simulink model "HA2_Active_Body_Control_stud"  (R2016a)
settings: Solver=VariableStepAuto  StartTime=0.0  StopTime=10  FixedStep=0.01  RelTol=1e-3
values from neighbouring files (symbols this model uses):
  A_cyl = pi*(D_kolben^2)/4    (= 0.000314159265359)    [Active_Body_Control_param_stud.m]
  alpha_K_va = 0.6    [Active_Body_Control_param_stud.m]
  bore_max = 20e-6    (= 2e-05)    [Active_Body_Control_param_stud.m]
  c_A = 19000    [Active_Body_Control_param_stud.m]
  c_R = 190500    [Active_Body_Control_param_stud.m]
  d = 59    [Active_Body_Control_param_stud.m]
  d_A = 1100    [Active_Body_Control_param_stud.m]
  delta_y_s = 0.005    [Active_Body_Control_param_stud.m]
  g = 9.81    [Active_Body_Control_param_stud.m]
  Km = 1    [Active_Body_Control_param_stud.m]
  L = 1e-5    (= 1e-05)    [Active_Body_Control_param_stud.m]
  m_A = 200    [Active_Body_Control_param_stud.m]
  m_R = 40    [Active_Body_Control_param_stud.m]
  m_va = 0.1    [Active_Body_Control_param_stud.m]
  P_pump = 150e5    (= 15000000)    [Active_Body_Control_param_stud.m]
  R = 1.2    [Active_Body_Control_param_stud.m]
  rho = 880    [Active_Body_Control_param_stud.m]
  s_max_va = 0.020    (= 0.02)    [Active_Body_Control_param_stud.m]
settings Model: Creator=da.klinder  LastModifiedBy=Jason
settings DataIOCC: LimitDataPoints=on  SaveFormat=Array  SignalLoggingSaveFormat=ModelDataLogs
settings OptimizationCC: ExpressionDepthLimit=2147483647
settings DebuggingCC: UnderspecifiedInitializationDetection=Classic  MergeDetectMultiDrivingBlocksExec=none  SolverPrmCheckMsg=warning  FcnCallInpInsideContextMsg=EnableAllAsWarning  StateNameClashWarn=warning
settings HardwareCC: ProdBitPerPointer=32  ProdLargestAtomicFloat=None  ProdIntDivRoundTo=Undefined  ProdEndianess=Unspecified  ProdWordSize=32  ProdHWDeviceType=32-bit Generic
settings ModelReferenceCC: PropagateSignalLabelsOutOfModel=off
settings GRTTargetCC: CombineOutputUpdateFcns=off  GRTInterface=on

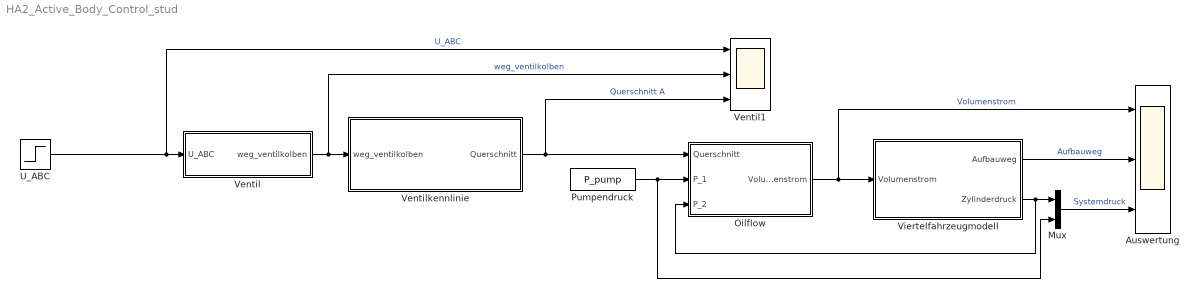
== system HA2_Active_Body_Control_stud ==
  Auswertung : Scope  NumInputPorts=3
  Mux : Mux  Inputs=2
  Oilflow : Subsystem
  Pumpendruck : Constant  Value=P_pump
  U_ABC : Step  Before=1  After=-1  SampleTime=0
  Ventil : Subsystem
  Ventil1 : Scope  NumInputPorts=3
  Ventilkennlinie : Subsystem
  Viertelfahrzeugmodell : Subsystem
  wires:
  Ventil/1(weg_ventilkolben) -> Ventilkennlinie/1(weg_ventilkolben), Ventil1/2  "weg_ventilkolben"
  Pumpendruck/1 -> Mux/2, Oilflow/2(P_1)
  Ventilkennlinie/1(Querschnitt) -> Ventil1/3, Oilflow/1(Querschnitt)  "Querschnitt A"
  Oilflow/1(Volumenstrom) -> Auswertung/1, Viertelfahrzeugmodell/1(Volumenstrom)  "Volumenstrom"
  Viertelfahrzeugmodell/2(Zylinderdruck) -> Mux/1, Oilflow/3(P_2)
  Mux/1 -> Auswertung/3  "Systemdruck"
  U_ABC/1 -> Ventil1/1, Ventil/1(U_ABC)  "U_ABC"
  Viertelfahrzeugmodell/1(Aufbauweg) -> Auswertung/2  "Aufbauweg"

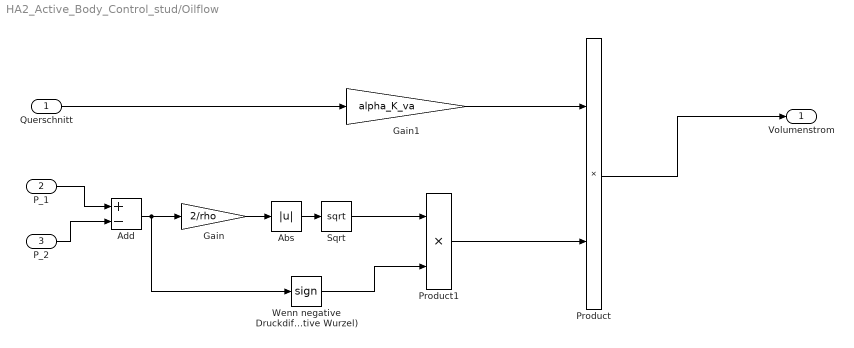
== system HA2_Active_Body_Control_stud/Oilflow ==
  Querschnitt : Inport
  P_1 : Inport  Port=2
  P_2 : Inport  Port=3
  Abs : Abs
  Add : Sum  Inputs=+-
  Gain : Gain  Gain=2/rho
  Gain1 : Gain  Gain=alpha_K_va
  Product : Product
  Product1 : Product
  Sqrt : Sqrt  SaturateOnIntegerOverflow=on
  "Wenn negative Druckdifferenz, dann auch negativer Volumenstrom (verhindert negative Wurzel)" : Signum
  Volumenstrom : Outport
  wires:
  P_1/1 -> Add/1
  P_2/1 -> Add/2
  Add/1 -> "Wenn negative Druckdifferenz, dann auch negativer Volumenstrom (verhindert negative Wurzel)"/1, Gain/1
  Gain/1 -> Abs/1
  Querschnitt/1 -> Gain1/1
  Product/1 -> Volumenstrom/1
  Abs/1 -> Sqrt/1
  Gain1/1 -> Product/1
  Sqrt/1 -> Product1/1
  "Wenn negative Druckdifferenz, dann auch negativer Volumenstrom (verhindert negative Wurzel)"/1 -> Product1/2
  Product1/1 -> Product/2

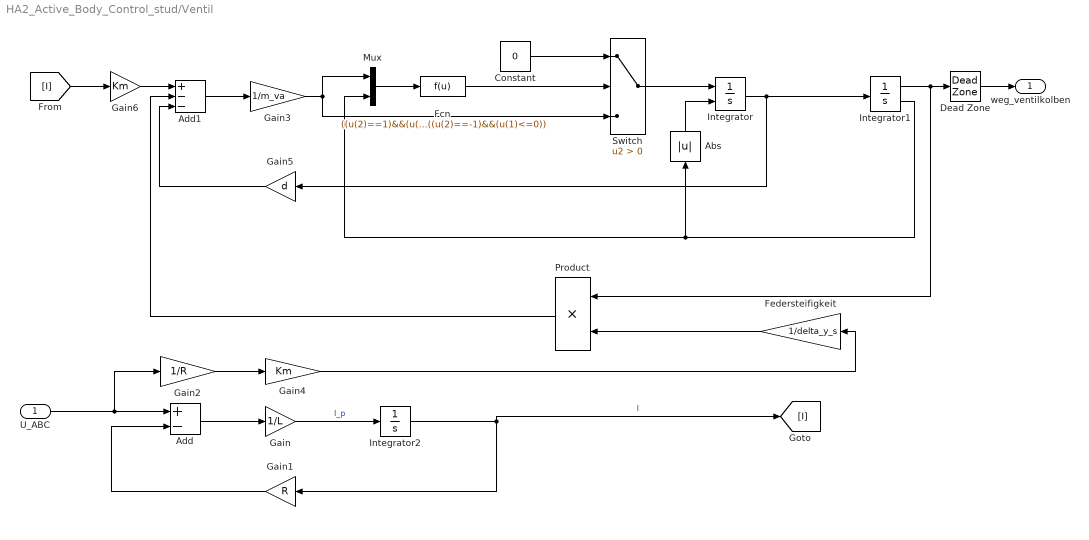
== system HA2_Active_Body_Control_stud/Ventil ==
  U_ABC : Inport
  Abs : Abs
  Add : Sum  Inputs=+-
  Add1 : Sum  Inputs=+--
  Constant : Constant  Value=0
  Dead Zone : DeadZone  SaturateOnIntegerOverflow=on
  Fcn : Fcn  Expr=((u(2)==1)&&(u(1)>=0))||((u(2)==-1)&&(u(1)<=0))
  Federsteifigkeit : Gain  Gain=1/delta_y_s
  Gain : Gain  Gain=1/L
  Gain1 : Gain  Gain=R
  Gain2 : Gain  Gain=1/R
  Gain3 : Gain  Gain=1/m_va
  Gain4 : Gain  Gain=Km
  Gain5 : Gain  Gain=d
  Gain6 : Gain  Gain=Km
  Integrator : Integrator  ExternalReset=rising
  Integrator1 : Integrator  LimitOutput=on  UpperSaturationLimit=s_max_va  LowerSaturationLimit=-s_max_va  ShowSaturationPort=on
  Integrator2 : Integrator
  Mux : Mux  Inputs=2
  Product : Product
  Switch : Switch  Criteria=u2 > Threshold
  weg_ventilkolben : Outport
  wires:
  Integrator/1 -> Gain5/1, Integrator1/1
  Integrator2/1 -> [I], Gain1/1  "I"
  Gain1/1 -> Add/2
  Add/1 -> Gain/1
  Gain/1 -> Integrator2/1  "I_p"
  Gain4/1 -> Federsteifigkeit/1
  Add1/1 -> Gain3/1
  Integrator1/1 -> Dead Zone/1, Product/1
  Gain5/1 -> Add1/3
  Federsteifigkeit/1 -> Product/2
  Product/1 -> Add1/2
  Gain2/1 -> Gain4/1
  [I] -> Gain6/1
  Gain6/1 -> Add1/1
  Constant/1 -> Switch/1
  Fcn/1 -> Switch/2
  Gain3/1 -> Mux/1, Switch/3
  Dead Zone/1 -> weg_ventilkolben/1
  Integrator1/2 -> Mux/2, Abs/1
  Mux/1 -> Fcn/1
  Switch/1 -> Integrator/1
  U_ABC/1 -> Gain2/1, Add/1
  Abs/1 -> Integrator/2

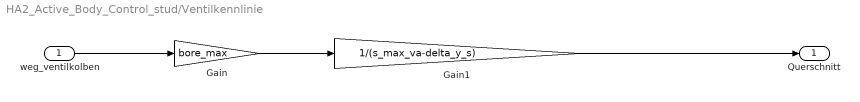
== system HA2_Active_Body_Control_stud/Ventilkennlinie ==
  weg_ventilkolben : Inport
  Gain : Gain  Gain=bore_max
  Gain1 : Gain  Gain=1/(s_max_va-delta_y_s)
  Querschnitt : Outport
  wires:
  weg_ventilkolben/1 -> Gain/1
  Gain/1 -> Gain1/1
  Gain1/1 -> Querschnitt/1

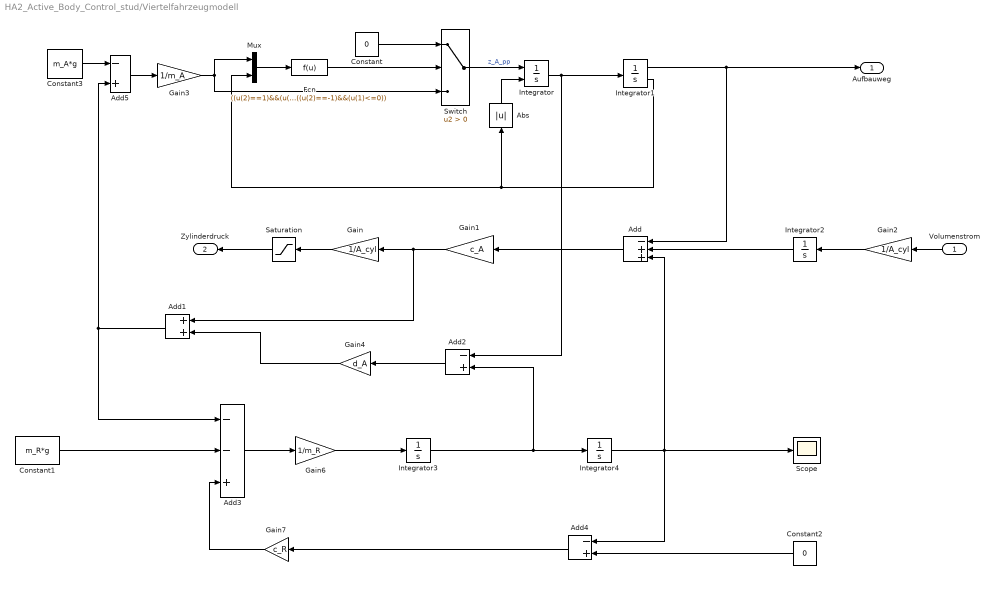
== system HA2_Active_Body_Control_stud/Viertelfahrzeugmodell ==
  Volumenstrom : Inport
  Abs : Abs
  Add : Sum  Inputs=-++
  Add1 : Sum
  Add2 : Sum  Inputs=-+
  Add3 : Sum  Inputs=--+
  Add4 : Sum  Inputs=-+
  Add5 : Sum  Inputs=-+
  Constant : Constant  Value=0
  Constant1 : Constant  Value=m_R*g
  Constant2 : Constant  Value=0
  Constant3 : Constant  Value=m_A*g
  Fcn : Fcn  Expr=((u(2)==1)&&(u(1)>=0))||((u(2)==-1)&&(u(1)<=0))
  Gain : Gain  Gain=1/A_cyl
  Gain1 : Gain  Gain=c_A
  Gain2 : Gain  Gain=1/A_cyl
  Gain3 : Gain  Gain=1/m_A
  Gain4 : Gain  Gain=d_A
  Gain6 : Gain  Gain=1/m_R
  Gain7 : Gain  Gain=c_R
  Integrator : Integrator  ExternalReset=rising
  Integrator1 : Integrator  LimitOutput=on  UpperSaturationLimit=s_max_va  LowerSaturationLimit=-s_max_va  ShowSaturationPort=on
  Integrator2 : Integrator
  Integrator3 : Integrator
  Integrator4 : Integrator
  Mux : Mux  Inputs=2
  Saturation : Saturate
  Scope : Scope
  Switch : Switch  Criteria=u2 > Threshold
  Aufbauweg : Outport
  Zylinderdruck : Outport  Port=2
  wires:
  Integrator1/2 -> Mux/2, Abs/1
  Mux/1 -> Fcn/1
  Integrator/1 -> Integrator1/1, Add2/1
  Abs/1 -> Integrator/2
  Add5/1 -> Gain3/1
  Switch/1 -> Integrator/1  "z_A_pp"
  Gain3/1 -> Mux/1, Switch/3
  Constant/1 -> Switch/1
  Fcn/1 -> Switch/2
  Saturation/1 -> Zylinderdruck/1
  Gain/1 -> Saturation/1
  Gain1/1 -> Add1/1, Gain/1
  Volumenstrom/1 -> Gain2/1
  Integrator2/1 -> Add/2
  Add/1 -> Gain1/1
  Gain2/1 -> Integrator2/1
  Gain4/1 -> Add1/2
  Add2/1 -> Gain4/1
  Constant1/1 -> Add3/2
  Add3/1 -> Gain6/1
  Gain6/1 -> Integrator3/1
  Integrator3/1 -> Add2/2, Integrator4/1
  Add4/1 -> Gain7/1
  Constant2/1 -> Add4/2
  Gain7/1 -> Add3/3
  Integrator4/1 -> Add4/1, Add/3, Scope/1
  Constant3/1 -> Add5/1
  Add1/1 -> Add5/2, Add3/1
  Integrator1/1 -> Add/1, Aufbauweg/1
